simulink model "CoTE_ThermDem"  (R2016b)
settings: configuration reference "CodeGenConfigSet" (kept outside this file)
settings Model: Creator=Colin  LastModifiedBy=Colin
settings ConfigSetRef: SourceLocation=Base Workspace

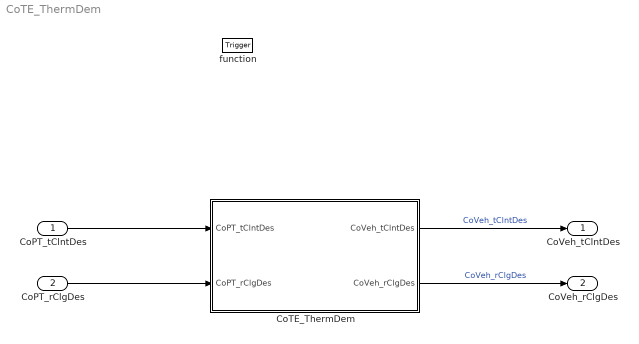
== system CoTE_ThermDem ==
  CoPT_tClntDes : Inport  Tag=deg  Description=Desired coolent temperature of the impulse rope  OutMin=-150  OutMax=150  OutDataTypeStr=Temp_deg
  CoPT_rClgDes : Inport  Tag=%  Description=Whole cool demand of the impulse rope for the ventilator  Port=2  OutMin=-300  OutMax=300  OutDataTypeStr=Prc_100_rate
  function : TriggerPort  TriggerType=function-call  VariantControl=Variant
  CoTE_ThermDem : Subsystem
  CoVeh_tClntDes : Outport  Tag=deg  Description=Desired coolant temperature  OutMin=-150  OutMax=150  OutDataTypeStr=Temp_deg
  CoVeh_rClgDes : Outport  Tag=%  Description=Desired relative air mass flow  Port=2  OutMin=-300  OutMax=300  OutDataTypeStr=Prc_100_rate
  wires:
  CoPT_tClntDes/1 -> CoTE_ThermDem/1(CoPT_tClntDes)
  CoTE_ThermDem/1(CoVeh_tClntDes) -> CoVeh_tClntDes/1  "CoVeh_tClntDes"
  CoPT_rClgDes/1 -> CoTE_ThermDem/2(CoPT_rClgDes)
  CoTE_ThermDem/2(CoVeh_rClgDes) -> CoVeh_rClgDes/1  "CoVeh_rClgDes"

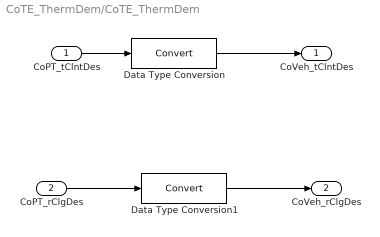
== system CoTE_ThermDem/CoTE_ThermDem ==
  CoPT_tClntDes : Inport
  CoPT_rClgDes : Inport  Port=2
  Data Type Conversion : DataTypeConversion
  Data Type Conversion1 : DataTypeConversion
  CoVeh_tClntDes : Outport
  CoVeh_rClgDes : Outport  Port=2
  wires:
  CoPT_tClntDes/1 -> Data Type Conversion/1
  Data Type Conversion/1 -> CoVeh_tClntDes/1
  CoPT_rClgDes/1 -> Data Type Conversion1/1
  Data Type Conversion1/1 -> CoVeh_rClgDes/1
